simulink model "sl_opspace"  (R2019b)
settings: Solver=VariableStepAuto  StartTime=0.0  StopTime=2  RelTol=1e-3  EnableMultiTasking=on
InitFcn:
  | fprintf('parameters initialized in InitFcn\n');
  | 
  | mdl_puma560
  | 
  | q = [0 pi/4 pi 0 -pi/4 0];
  | TE = p560.fkine(q);
  | Sf = TE.R
  | 
  | % edit next 2 lines to change compliant motion axes
  | %  1 = freespace controlled motion
  | %  0 = constrained compliant motion
  | 
  | sigma_f = diag([1 1 0]);  % translation
  | sigma_t = diag([1 1 1]);  % rotation
  | 
  | 
  | 
  | omega = blkdiag( Sf'*sigma_f*Sf, Sf'*sigma_t*Sf)
  | omega_tilde = blkdiag( Sf'*(eye(3,3)-sigma_f)*Sf, Sf'*(eye(3,3)-sigma_t)*Sf)
values from neighbouring files (symbols this model uses):
  qn = [0 -pi/4 0 0 -pi/4 0]    [Model_210F.m]    (also in Model_210F_old.m; WorkspContrPointToPoint.mat = [0 0.785398163397 3.14159265359 0 0.785398163397 0]; matlab.mat = [0 0.785398163397 3.14159265359 0 0.785398163397 0]; timings.mat = [0 0.785398163397 3.14159265359 0 0.785398163397 0])
undefined symbols (not defined in the file or in its folder): cinertia, nofriction, p560, robot, transl, troty
libraries: roblocks x8
settings Model: Creator=corkep  LastModifiedBy=Karl
settings DataIOCC: LimitDataPoints=on  SaveFormat=Array  TimeSaveName=t  OutputSaveName=y  ReturnWorkspaceOutputsName=opspace
settings OptimizationCC: LifeSpan=inf
settings DebuggingCC: AllowSymbolicDim=off  SFUnexpectedBacktrackingDiag=warning  SFNoUnconditionalDefaultTransitionDiag=warning  SFExecutionAtInitializationDiag=none  ArithmeticOperatorsInVariantConditions=warning
settings ModelReferenceCC: PropagateSignalLabelsOutOfModel=off
settings SFSimCC: SimUseLocalCustomCode=off  CustomCodeUndefinedFunction=UseInterfaceOnly
settings RTWCC: RTWUseLocalCustomCode=off
settings CodeAppCC: StateflowObjectComments=on
settings GRTTargetCC: TargetLangStandard=C89/C90 (ANSI)
settings ConfigComp: CovMetricSettings=dw  CovHtmlReporting=on  CovSaveCumulativeToWorkspaceVar=on  CovSaveSingleToWorkspaceVar=on  CovExternalEMLEnable=off

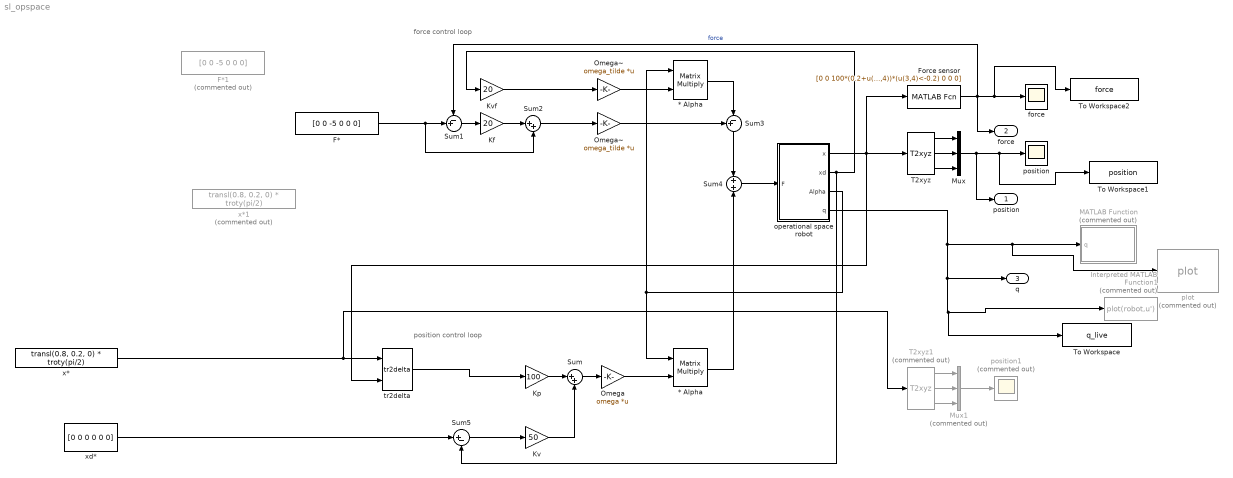
== system sl_opspace ==
  note: position control loop
  note: force control loop
  * Alpha : Product  Multiplication=Matrix(*)
  "* Alpha " : Product  Multiplication=Matrix(*)
  F* : Constant  Value=[0 0 -5 0 0 0]
  F*1 : Constant  Commented=on  Value=[0 0 -5 0 0 0]
  Force sensor : MATLABFcn  MATLABFcn=[0 0 100*(0.2+u(3,4))*(u(3,4)<-0.2) 0 0 0]
  Interpreted MATLAB Function1 : MATLABFcn  Commented=on  MATLABFcn=plot(robot,u')  OutputDimensions=0
  Kf : Gain  Gain=20
  Kp : Gain  Gain=100
  Kv : Gain  Gain=50
  Kvf : Gain  Gain=20
  MATLAB Function : MATLAB Function  Commented=on  TreatAsAtomicUnit=on
  Mux : Mux  Inputs=3
  Mux1 : Mux  Commented=on  Inputs=3
  Omega : Gain  Gain=omega  Multiplication=Matrix(K*u)
  Omega~ : Gain  Gain=omega_tilde  Multiplication=Matrix(K*u)
  "Omega~ " : Gain  Gain=omega_tilde  Multiplication=Matrix(K*u)
  Sum : Sum  Inputs=|++
  Sum1 : Sum  Inputs=-+|
  Sum2 : Sum  Inputs=|++
  Sum3 : Sum  Inputs=+-|
  Sum4 : Sum  Inputs=+|+
  Sum5 : Sum  Inputs=|+-
  T2xyz : roblocks/Toolbox/T2xyz
  T2xyz1 : roblocks/Toolbox/T2xyz  Commented=on
  To Workspace : ToWorkspace  VariableName=q_live  SaveFormat=Timeseries  SampleTime=-1
  To Workspace1 : ToWorkspace  VariableName=position  SaveFormat=Timeseries  SampleTime=-1
  To Workspace2 : ToWorkspace  VariableName=force  SaveFormat=Timeseries  SampleTime=-1
  force : Scope
  operational space robot : Subsystem  mask{robot=nofriction(p560), q0=qn}
      mask prompts: q0 "Initial joint angles"
  plot : roblocks/Arm/plot  Commented=on  robot=p560  fps=20  holdplot=on
  position : Scope
  position1 : Scope  Commented=on
  tr2delta : roblocks/Toolbox/tr2delta
  x* : Constant  Value=transl(0.8, 0.2, 0) * troty(pi/2)
  x*1 : Constant  Commented=on  Value=transl(0.8, 0.2, 0) * troty(pi/2)
  xd* : Constant  Value=[0 0 0 0 0 0]
  "position " : Outport
  "force " : Outport  Port=2
  q : Outport  Port=3
  wires:
  x*/1 -> tr2delta/1, T2xyz1/1
  operational space robot/1(x) -> tr2delta/2, T2xyz/1, Force sensor/1
  operational space robot/3(Alpha) -> * Alpha/1, "* Alpha "/1
  Sum/1 -> Omega/1
  Kp/1 -> Sum/1
  Kv/1 -> Sum/2
  operational space robot/2(xd) -> Kvf/1, Sum5/2
  Force sensor/1 -> "force "/1, To Workspace2/1, force/1, Sum1/1  "force"
  F*/1 -> Sum2/2, Sum1/2
  Sum1/1 -> Kf/1
  Kf/1 -> Sum2/1
  Kvf/1 -> Omega~/1
  Sum2/1 -> "Omega~ "/1
  Omega~/1 -> * Alpha/2
  * Alpha/1 -> Sum3/2
  "Omega~ "/1 -> Sum3/1
  Sum3/1 -> Sum4/1
  "* Alpha "/1 -> Sum4/2
  Omega/1 -> "* Alpha "/2
  xd*/1 -> Sum5/1
  Sum5/1 -> Kv/1
  Sum4/1 -> operational space robot/1(F)
  T2xyz/1 -> Mux/1
  T2xyz/2 -> Mux/2
  T2xyz/3 -> Mux/3
  Mux/1 -> "position "/1, To Workspace1/1, position/1
  operational space robot/4(q) -> q/1, To Workspace/1, Interpreted MATLAB Function1/1, plot/1, MATLAB Function/1(q)
  T2xyz1/1 -> Mux1/1
  T2xyz1/2 -> Mux1/2
  T2xyz1/3 -> Mux1/3
  Mux1/1 -> position1/1
  tr2delta/1 -> Kp/1

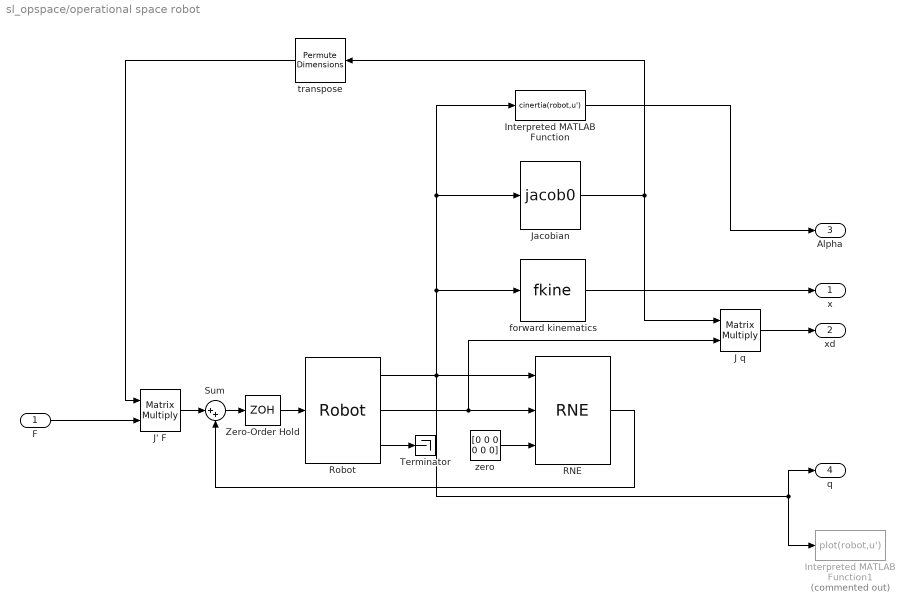
== system sl_opspace/operational space robot ==
  F : Inport
  Interpreted MATLAB Function : MATLABFcn  MATLABFcn=cinertia(robot,u')  OutputDimensions=[6 6]  Output1D=off
  Interpreted MATLAB Function1 : MATLABFcn  Commented=on  MATLABFcn=plot(robot,u')  OutputDimensions=0
  J q : Product  Multiplication=Matrix(*)
  J' F : Product  Multiplication=Matrix(*)
  Jacobian : roblocks/Arm/jacob0   robot=robot
  RNE : roblocks/Arm/RNE  robot=robot  grav=[0 0 9.81]
  Robot : roblocks/Arm/Robot  robot=robot  q0=q0
  Sum : Sum  Inputs=|++
  Terminator : Terminator
  Zero-Order Hold : ZeroOrderHold  SampleTime=5e-3
  forward kinematics : roblocks/Arm/fkine  robot=robot
  transpose : PermuteDimensions
  zero : Constant  Value=[0 0 0 0 0 0]
  x : Outport
  xd : Outport  Port=2
  Alpha : Outport  Port=3
  q : Outport  Port=4
  wires:
  Interpreted MATLAB Function/1 -> Alpha/1
  Zero-Order Hold/1 -> Robot/1
  Sum/1 -> Zero-Order Hold/1
  F/1 -> J' F/2
  transpose/1 -> J' F/1
  J' F/1 -> Sum/1
  RNE/1 -> Sum/2
  zero/1 -> RNE/3
  Robot/3 -> Terminator/1
  Robot/2 -> J q/2, RNE/2
  Robot/1 -> forward kinematics/1, Interpreted MATLAB Function/1, Jacobian/1, RNE/1, q/1, Interpreted MATLAB Function1/1
  forward kinematics/1 -> x/1
  J q/1 -> xd/1
  Jacobian/1 -> transpose/1, J q/1

== matlab function sl_opspace/MATLAB Function ==
  data: q input
function  fcn(q)

p560.plot(q)
